simulink model "mass_diff"  (Simulink 7.9)
settings: Solver=ode3  StartTime=0.0  StopTime=10.0  RelTol=1e-3
libraries: simulink x1
settings Model: Creator=dAN  LastModifiedBy=dAN

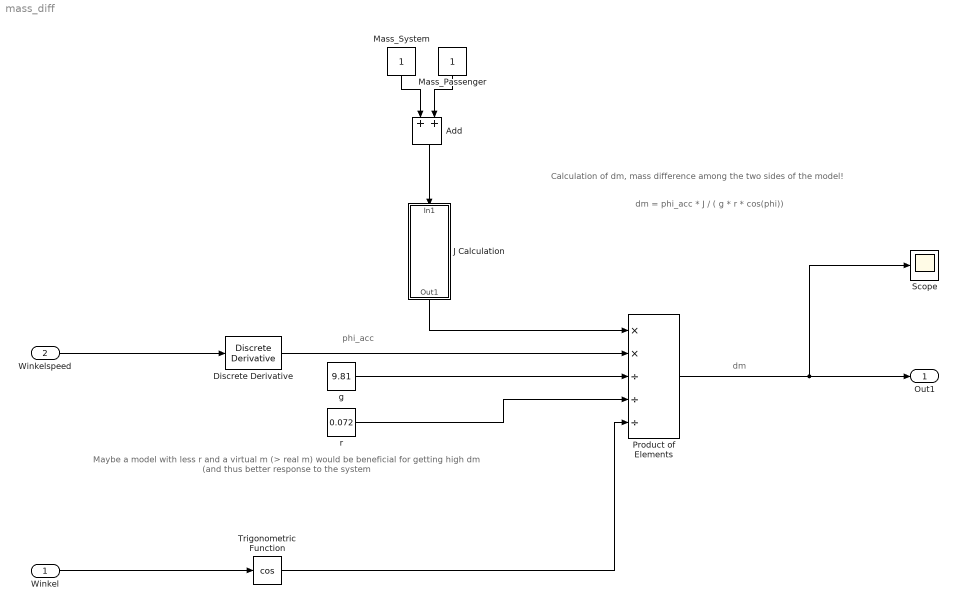
== system mass_diff ==
  note: Calculation of dm, mass difference among the two sides of the model!
  note: dm = phi_acc * J / ( g * r * cos(phi))
  note: dm
  note: phi_acc
  note: Maybe a model with less r and a virtual m (> real m) would be beneficial for getting high dm (and thus better response to the system
  Winkel : Inport
  Winkelspeed : Inport  Port=2
  Add : Sum
  Discrete Derivative : simulink/Discrete/Discrete Derivative  gainval=1.0  ICPrevScaledInput=0.0  InputProcessing=Inherited  OutMin=[]  OutMax=[]  OutDataType=fixdt(1, 16)  OutScaling=2^-10  DoSatur=off
  J Calculation : Subsystem
  Mass_Passenger : Constant
  Mass_System : Constant
  Product of Elements : Product  Inputs=**///
  Scope : Scope
  Trigonometric Function : Trigonometry  Operator=cos
  g : Constant  Value=9.81
  r : Constant  Value=0.072
  Out1 : Outport
  wires:
  Mass_Passenger/1 -> Add/2
  Mass_System/1 -> Add/1
  Add/1 -> J Calculation/1(In1)
  Product of Elements/1 -> Out1/1, Scope/1
  J Calculation/1(Out1) -> Product of Elements/1
  Discrete Derivative/1 -> Product of Elements/2
  g/1 -> Product of Elements/3
  r/1 -> Product of Elements/4
  Trigonometric Function/1 -> Product of Elements/5
  Winkelspeed/1 -> Discrete Derivative/1
  Winkel/1 -> Trigonometric Function/1

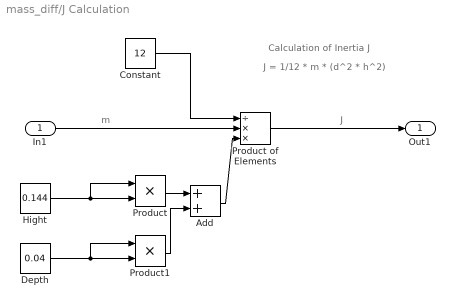
== system mass_diff/J Calculation ==
  note: Calculation of Inertia J
  note: J = 1/12 * m * (d^2 * h^2)
  note: J
  note: m
  In1 : Inport
  Add : Sum
  Constant : Constant  Value=12
  Depth : Constant  Value=0.04
  Hight : Constant  Value=0.144
  Product : Product  RndMeth=Zero
  Product of Elements : Product  Inputs=/**
  Product1 : Product  RndMeth=Zero
  Out1 : Outport
  wires:
  Constant/1 -> Product of Elements/1
  In1/1 -> Product of Elements/2
  Depth/1 -> Product1/1, Product1/2
  Hight/1 -> Product/1, Product/2
  Add/1 -> Product of Elements/3
  Product/1 -> Add/1
  Product1/1 -> Add/2
  Product of Elements/1 -> Out1/1
